simulink model "Vizualize_Measurement"  (R2018b)
settings: Solver=VariableStepAuto  StartTime=0  StopTime=(31+29+31+30+31+30+31+14)*24*3600  RelTol=1e-3  EnableMultiTasking=on
libraries: carnot x16
settings Model: SimulationMode=accelerator  Creator=U_13.adm_zivi  LastModifiedBy=drhf
settings DataIOCC: SaveFormat=Array  SignalLoggingSaveFormat=ModelDataLogs  SaveOutput=off  SignalLogging=off  SaveTime=off
settings OptimizationCC: ExpressionDepthLimit=2147483647  LifeSpan=inf
settings DebuggingCC: UnderspecifiedInitializationDetection=Classic  MergeDetectMultiDrivingBlocksExec=none  SolverPrmCheckMsg=warning  FcnCallInpInsideContextMsg=warning  StateNameClashWarn=warning  SFUnexpectedBacktrackingDiag=warning  SFNoUnconditionalDefaultTransitionDiag=warning  SFExecutionAtInitializationDiag=none
settings HardwareCC: ProdBitPerPointer=32  ProdBitPerSizeT=32  ProdBitPerPtrDiffT=32  ProdLargestAtomicFloat=None  ProdIntDivRoundTo=Undefined  ProdEndianess=Unspecified  ProdWordSize=32  ProdHWDeviceType=32-bit Generic
settings ModelReferenceCC: PropagateSignalLabelsOutOfModel=off
settings SFSimCC: SimUseLocalCustomCode=off
settings RTWCC: RTWUseLocalCustomCode=off
settings CodeAppCC: StateflowObjectComments=on
settings GRTTargetCC: TargetLangStandard=C89/C90 (ANSI)  GeneratePreprocessorConditionals=Disable all  CombineOutputUpdateFcns=off  GRTInterface=on
settings ConfigComp: CovMetricSettings=dw  CovHtmlReporting=on  CovSaveCumulativeToWorkspaceVar=on  CovSaveSingleToWorkspaceVar=on  CovExternalEMLEnable=off

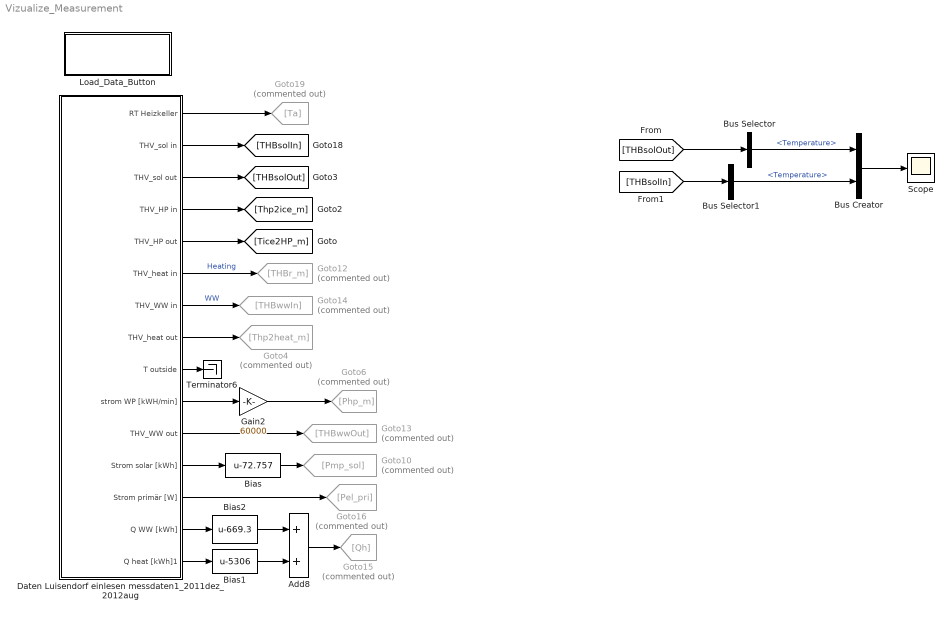
== system Vizualize_Measurement ==
  Add8 : Sum
  Bias : Bias  Bias=-72.757
  Bias1 : Bias  Bias=-5306
  Bias2 : Bias  Bias=-669.3
  Bus Creator : BusCreator  Inputs=2
  Bus Selector : BusSelector  OutputSignals=Temperature
  Bus Selector1 : BusSelector  OutputSignals=Temperature
  Daten Luisendorf einlesen messdaten1_2011dez_2012aug : Subsystem
  Gain2 : Gain  Gain=60000
  Goto10 : Goto  Commented=on  GotoTag=Pmp_sol
  Goto12 : Goto  Commented=on  GotoTag=THBr_m
  Goto13 : Goto  Commented=on  GotoTag=THBwwOut
  Goto14 : Goto  Commented=on  GotoTag=THBwwIn
  Goto15 : Goto  Commented=on  GotoTag=Qh
  Goto16 : Goto  Commented=on  GotoTag=Pel_pri
  Goto19 : Goto  Commented=on  GotoTag=Ta
  Goto4 : Goto  Commented=on  GotoTag=Thp2heat_m
  Goto6 : Goto  Commented=on  GotoTag=Php_m
  Load_Data_Button : Subsystem
      settings: OpenFcn=|
      | [filename, pathname, filterindex] = ...
      |    uigetfile( {'*.mat','MAT-files (*.mat)'; ...
      |    '*.*',  'All Files (*.*)'},  'Pick a data file');
      | 
      | if (filterindex > 0)
      |    load(filename)
      | end
      mask Display: disp('double click \nto load data')
  Scope : Scope
  Terminator6 : Terminator
  wires:
  Daten Luisendorf einlesen messdaten1_2011dez_2012aug/5(THV_HP out) -> [Tice2HP_m]
  Bus Creator/1 -> Scope/1
  Daten Luisendorf einlesen messdaten1_2011dez_2012aug/6(THV_heat in) -> Goto12/1  "Heating"
  Daten Luisendorf einlesen messdaten1_2011dez_2012aug/7(THV_WW in) -> Goto14/1  "WW"
  Daten Luisendorf einlesen messdaten1_2011dez_2012aug/4(THV_HP in) -> [Thp2ice_m]
  Daten Luisendorf einlesen messdaten1_2011dez_2012aug/10(strom WP [kWH/min]) -> Gain2/1
  Daten Luisendorf einlesen messdaten1_2011dez_2012aug/8(THV_heat out) -> Goto4/1
  Daten Luisendorf einlesen messdaten1_2011dez_2012aug/11(THV_WW out) -> Goto13/1
  Daten Luisendorf einlesen messdaten1_2011dez_2012aug/12(Strom solar [kWh]) -> Bias/1
  Bias2/1 -> Add8/1
  Daten Luisendorf einlesen messdaten1_2011dez_2012aug/14(Q WW [kWh]) -> Bias2/1
  Daten Luisendorf einlesen messdaten1_2011dez_2012aug/15(Q heat [kWh]1) -> Bias1/1
  Daten Luisendorf einlesen messdaten1_2011dez_2012aug/9(T outside) -> Terminator6/1
  Daten Luisendorf einlesen messdaten1_2011dez_2012aug/3(THV_sol out) -> [THBsolOut]
  Gain2/1 -> Goto6/1
  Bias/1 -> Goto10/1
  Bias1/1 -> Add8/2
  Add8/1 -> Goto15/1
  Daten Luisendorf einlesen messdaten1_2011dez_2012aug/13(Strom primär [W]) -> Goto16/1
  Daten Luisendorf einlesen messdaten1_2011dez_2012aug/2(THV_sol in) -> [THBsolIn]
  Daten Luisendorf einlesen messdaten1_2011dez_2012aug/1(RT Heizkeller) -> Goto19/1
  [THBsolOut] -> Bus Selector/1
  [THBsolIn] -> Bus Selector1/1
  Bus Selector/1 -> Bus Creator/1  "<Temperature>"
  Bus Selector1/1 -> Bus Creator/2  "<Temperature>"

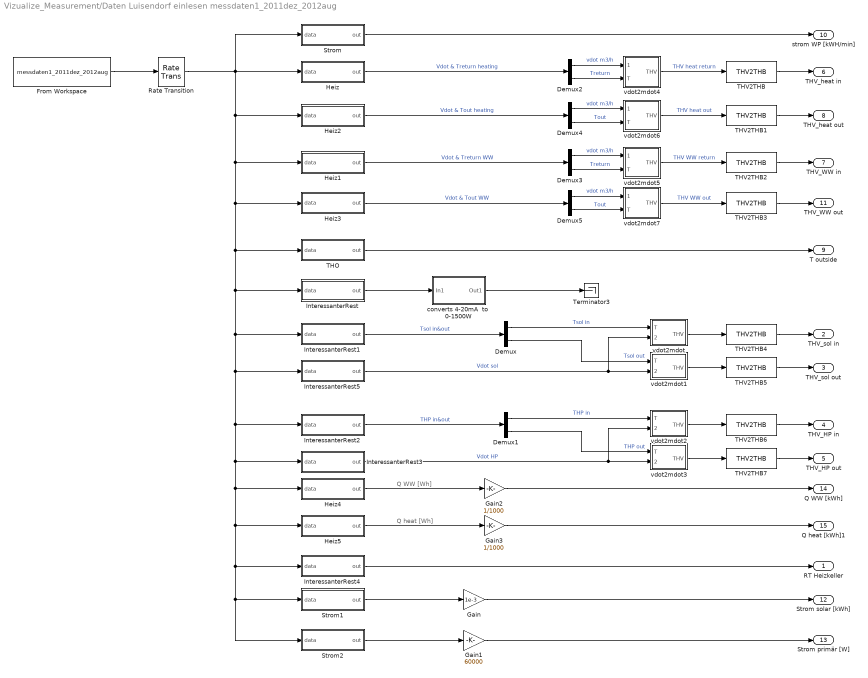
== system Vizualize_Measurement/Daten Luisendorf einlesen messdaten1_2011dez_2012aug ==
  note: Q WW [Wh]
  note: Q heat [Wh]
  Demux{,1..5} (6 alike) : Demux  Outputs=2
  From Workspace : FromWorkspace  VariableName=messdaten1_2011dez_2012aug  SampleTime=60  Interpolate=off  OutputAfterFinalValue=Holding final value
  Gain : Gain  Gain=1e-3
  Gain1 : Gain  Gain=60000
  Gain2 : Gain  Gain=1/1000
  Gain3 : Gain  Gain=1/1000
  Heiz : Subsystem  mask(Selector Messdaten Viessmann){a1=off, a2=off, a3=on, a4=off, a5=on, a6=off, a7=off, a8=off, a9=off, a10=off}
      mask prompts: a1 "Heizkreis_Wh [NONE]"; a2 "Heizkreis_m3 [NONE]"; a3 "Heizkreis_m3/h [NONE]"; a4 "Heizkreis_Tflow [NONE]"; a5 "Heizkreis_Treturn [NONE]"; a6 "TWW+Zirkulation_Wh [NONE]"; a7 "TWW+Zirkulation_m3 [NONE]"; a8 "TWW+Zirkulation_m3/h [NONE]"; a9 "TWW+Zirkulation_Tflow [NONE]"; a10 "TWW+Zirkulation_Treturn [NONE]"
      mask help:
      | Wählt die Messdaten der Viessmann Eisspeicher Anlage aus.
      | Daten der Messungen:
      | Dezember 2011 - August 2012
      mask init:
      | v=[];
      | if (a1)  v = [4];     end
      | if (a2)  v = [v 5];     end
      | if (a3)  v = [v 6];    end
      | if (a4)  v = [v 7];    end
      | if (a5)  v = [v 8];    end
      | if (a6)  v = [v 29];    end
      | if (a7)  v = [v 30];    end
      | if (a8)  v = [v 31];    end
      | if (a9)  v = [v 32];    end
      | if (a10)  v = [v 33];    end
      | if (~numel(v)) v = [6]; end
  Heiz1 : Subsystem  mask(Selector Messdaten Viessmann){a1=off, a2=off, a3=off, a4=off, a5=off, a6=off, a7=off, a8=on, a9=off, a10=on}
      mask prompts: a1 "Heizkreis_Wh [NONE]"; a2 "Heizkreis_m3 [NONE]"; a3 "Heizkreis_m3/h [NONE]"; a4 "Heizkreis_Tflow [NONE]"; a5 "Heizkreis_Treturn [NONE]"; a6 "TWW+Zirkulation_Wh [NONE]"; a7 "TWW+Zirkulation_m3 [NONE]"; a8 "TWW+Zirkulation_m3/h [NONE]"; a9 "TWW+Zirkulation_Tflow [NONE]"; a10 "TWW+Zirkulation_Treturn [NONE]"
      mask help:
      | Wählt die Messdaten der Viessmann Eisspeicher Anlage aus.
      | Daten der Messungen:
      | Dezember 2011 - August 2012
      mask init: same as Vizualize_Measurement/Daten Luisendorf einlesen messdaten1_2011dez_2012aug/Heiz
  Heiz2 : Subsystem  mask(Selector Messdaten Viessmann){a1=off, a2=off, a3=on, a4=on, a5=off, a6=off, a7=off, a8=off, a9=off, a10=off}
      mask prompts: a1 "Heizkreis_Wh [NONE]"; a2 "Heizkreis_m3 [NONE]"; a3 "Heizkreis_m3/h [NONE]"; a4 "Heizkreis_Tflow [NONE]"; a5 "Heizkreis_Treturn [NONE]"; a6 "TWW+Zirkulation_Wh [NONE]"; a7 "TWW+Zirkulation_m3 [NONE]"; a8 "TWW+Zirkulation_m3/h [NONE]"; a9 "TWW+Zirkulation_Tflow [NONE]"; a10 "TWW+Zirkulation_Treturn [NONE]"
      mask help:
      | Wählt die Messdaten der Viessmann Eisspeicher Anlage aus.
      | Daten der Messungen:
      | Dezember 2011 - August 2012
      mask init: same as Vizualize_Measurement/Daten Luisendorf einlesen messdaten1_2011dez_2012aug/Heiz
  Heiz3 : Subsystem  mask(Selector Messdaten Viessmann){a1=off, a2=off, a3=off, a4=off, a5=off, a6=off, a7=off, a8=on, a9=on, a10=off}
      mask prompts: a1 "Heizkreis_Wh [NONE]"; a2 "Heizkreis_m3 [NONE]"; a3 "Heizkreis_m3/h [NONE]"; a4 "Heizkreis_Tflow [NONE]"; a5 "Heizkreis_Treturn [NONE]"; a6 "TWW+Zirkulation_Wh [NONE]"; a7 "TWW+Zirkulation_m3 [NONE]"; a8 "TWW+Zirkulation_m3/h [NONE]"; a9 "TWW+Zirkulation_Tflow [NONE]"; a10 "TWW+Zirkulation_Treturn [NONE]"
      mask help:
      | Wählt die Messdaten der Viessmann Eisspeicher Anlage aus.
      | Daten der Messungen:
      | Dezember 2011 - August 2012
      mask init: same as Vizualize_Measurement/Daten Luisendorf einlesen messdaten1_2011dez_2012aug/Heiz
  Heiz4 : Subsystem  mask(Selector Messdaten Viessmann){a1=off, a2=off, a3=off, a4=off, a5=off, a6=on, a7=off, a8=off, a9=off, a10=off}
      mask prompts: a1 "Heizkreis_Wh [NONE]"; a2 "Heizkreis_m3 [NONE]"; a3 "Heizkreis_m3/h [NONE]"; a4 "Heizkreis_Tflow [NONE]"; a5 "Heizkreis_Treturn [NONE]"; a6 "TWW+Zirkulation_Wh [NONE]"; a7 "TWW+Zirkulation_m3 [NONE]"; a8 "TWW+Zirkulation_m3/h [NONE]"; a9 "TWW+Zirkulation_Tflow [NONE]"; a10 "TWW+Zirkulation_Treturn [NONE]"
      mask help:
      | Wählt die Messdaten der Viessmann Eisspeicher Anlage aus.
      | Daten der Messungen:
      | Dezember 2011 - August 2012
      mask init: same as Vizualize_Measurement/Daten Luisendorf einlesen messdaten1_2011dez_2012aug/Heiz
  Heiz5 : Subsystem  mask(Selector Messdaten Viessmann){a1=on, a2=off, a3=off, a4=off, a5=off, a6=off, a7=off, a8=off, a9=off, a10=off}
      mask prompts: a1 "Heizkreis_Wh [NONE]"; a2 "Heizkreis_m3 [NONE]"; a3 "Heizkreis_m3/h [NONE]"; a4 "Heizkreis_Tflow [NONE]"; a5 "Heizkreis_Treturn [NONE]"; a6 "TWW+Zirkulation_Wh [NONE]"; a7 "TWW+Zirkulation_m3 [NONE]"; a8 "TWW+Zirkulation_m3/h [NONE]"; a9 "TWW+Zirkulation_Tflow [NONE]"; a10 "TWW+Zirkulation_Treturn [NONE]"
      mask help:
      | Wählt die Messdaten der Viessmann Eisspeicher Anlage aus.
      | Daten der Messungen:
      | Dezember 2011 - August 2012
      mask init: same as Vizualize_Measurement/Daten Luisendorf einlesen messdaten1_2011dez_2012aug/Heiz
  InteressanterRest : Subsystem  mask(Selector Messdaten Viessmann){a1=on, a2=off, a3=off, a4=off, a5=off, a6=off, a7=off, a8=off, a9=off, a10=off, a11=off, a12=off, a13=off, a14=off}
      mask prompts: a1 "Einstrahlung [Ampere 4-20mA=0-1500W]"; a2 "Resol  Sol-Eis VL [Celsius]"; a3 "Resol Eis-WP [m^3]"; a4 "Resol Eis-WP RL [Celsius]"; a5 "Resol Eis-WP VL [Celsius]"; a6 "Resol Sol-Eis [m^3]"; a7 "Resol Sol-Eis RL [Celsius]"; a8 "Resol Sol-WP [m^3]"; a9 "Resol Sol-WP RL [Celsius]"; a10 "Resol Sol-WP VL [Celsius]"; a11 "RT Heizkeller [Celsius]"; a12 "Ventil R2_UmschKol [Volt]"; a13 "Ventil_R3_SolPumpe [Volt]"; a14 "Ventil_R4_UmschSpe [Volt]"
      mask help:
      | Wählt die Messdaten der Viessmann Eisspeicher Anlage aus.
      | Daten der Messungen:
      | Dezember 2011 - August 2012
      mask init:
      | v=[];
      | if (a1)  v = [3];     end
      | if (a2)  v = [v 9];     end
      | if (a3)  v = [v 10];    end
      | if (a4)  v = [v 11];    end
      | if (a5)  v = [v 12];    end
      | if (a6)  v = [v 13];    end
      | if (a7)  v = [v 14];     end
      | if (a8)  v = [v 15];     end
      | if (a9)  v = [v 16];    end
      | if (a10)  v = [v 17];    end
      | if (a11)  v = [v 18];    end
      | if (a12)  v = [v 34];    end
      | if (a13)  v = [v 35];     end
      | if (a14)  v = [v 36];     end
      | if (~numel(v)) v = [6]; end
  InteressanterRest1 : Subsystem  mask(Selector Messdaten Viessmann){a1=off, a2=on, a3=off, a4=off, a5=off, a6=off, a7=on, a8=off, a9=off, a10=off, a11=off, a12=off, a13=off, a14=off}
      mask prompts: a1 "Einstrahlung [Ampere 4-20mA=0-1500W]"; a2 "Resol  Sol-Eis VL [Celsius]"; a3 "Resol Eis-WP [m^3]"; a4 "Resol Eis-WP RL [Celsius]"; a5 "Resol Eis-WP VL [Celsius]"; a6 "Resol Sol-Eis [m^3]"; a7 "Resol Sol-Eis RL [Celsius]"; a8 "Resol Sol-WP [m^3]"; a9 "Resol Sol-WP RL [Celsius]"; a10 "Resol Sol-WP VL [Celsius]"; a11 "RT Heizkeller [Celsius]"; a12 "Ventil R2_UmschKol [Volt]"; a13 "Ventil_R3_SolPumpe [Volt]"; a14 "Ventil_R4_UmschSpe [Volt]"
      mask help:
      | Wählt die Messdaten der Viessmann Eisspeicher Anlage aus.
      | Daten der Messungen:
      | Dezember 2011 - August 2012
      mask init: same as Vizualize_Measurement/Daten Luisendorf einlesen messdaten1_2011dez_2012aug/InteressanterRest
  InteressanterRest2 : Subsystem  mask(Selector Messdaten Viessmann){a1=off, a2=off, a3=off, a4=on, a5=on, a6=off, a7=off, a8=off, a9=off, a10=off, a11=off, a12=off, a13=off, a14=off}
      mask prompts: a1 "Einstrahlung [Ampere 4-20mA=0-1500W]"; a2 "Resol  Sol-Eis VL [Celsius]"; a3 "Resol Eis-WP [m^3]"; a4 "Resol Eis-WP RL [Celsius]"; a5 "Resol Eis-WP VL [Celsius]"; a6 "Resol Sol-Eis [m^3]"; a7 "Resol Sol-Eis RL [Celsius]"; a8 "Resol Sol-WP [m^3]"; a9 "Resol Sol-WP RL [Celsius]"; a10 "Resol Sol-WP VL [Celsius]"; a11 "RT Heizkeller [Celsius]"; a12 "Ventil R2_UmschKol [Volt]"; a13 "Ventil_R3_SolPumpe [Volt]"; a14 "Ventil_R4_UmschSpe [Volt]"
      mask help:
      | Wählt die Messdaten der Viessmann Eisspeicher Anlage aus.
      | Daten der Messungen:
      | Dezember 2011 - August 2012
      mask init: same as Vizualize_Measurement/Daten Luisendorf einlesen messdaten1_2011dez_2012aug/InteressanterRest
  InteressanterRest3 : Subsystem  mask(Selector Messdaten Viessmann){a1=off, a2=off, a3=on, a4=off, a5=off, a6=off, a7=off, a8=off, a9=off, a10=off, a11=off, a12=off, a13=off, a14=off}
      mask prompts: a1 "Einstrahlung [Ampere 4-20mA=0-1500W]"; a2 "Resol  Sol-Eis VL [Celsius]"; a3 "Resol Eis-WP [m^3]"; a4 "Resol Eis-WP RL [Celsius]"; a5 "Resol Eis-WP VL [Celsius]"; a6 "Resol Sol-Eis [m^3]"; a7 "Resol Sol-Eis RL [Celsius]"; a8 "Resol Sol-WP [m^3]"; a9 "Resol Sol-WP RL [Celsius]"; a10 "Resol Sol-WP VL [Celsius]"; a11 "RT Heizkeller [Celsius]"; a12 "Ventil R2_UmschKol [Volt]"; a13 "Ventil_R3_SolPumpe [Volt]"; a14 "Ventil_R4_UmschSpe [Volt]"
      mask help:
      | Wählt die Messdaten der Viessmann Eisspeicher Anlage aus.
      | Daten der Messungen:
      | Dezember 2011 - August 2012
      mask init: same as Vizualize_Measurement/Daten Luisendorf einlesen messdaten1_2011dez_2012aug/InteressanterRest
  InteressanterRest4 : Subsystem  mask(Selector Messdaten Viessmann){a1=off, a2=off, a3=off, a4=off, a5=off, a6=off, a7=off, a8=off, a9=off, a10=off, a11=on, a12=off, a13=off, a14=off}
      mask prompts: a1 "Einstrahlung [Ampere 4-20mA=0-1500W]"; a2 "Resol  Sol-Eis VL [Celsius]"; a3 "Resol Eis-WP [m^3]"; a4 "Resol Eis-WP RL [Celsius]"; a5 "Resol Eis-WP VL [Celsius]"; a6 "Resol Sol-Eis [m^3]"; a7 "Resol Sol-Eis RL [Celsius]"; a8 "Resol Sol-WP [m^3]"; a9 "Resol Sol-WP RL [Celsius]"; a10 "Resol Sol-WP VL [Celsius]"; a11 "RT Heizkeller [Celsius]"; a12 "Ventil R2_UmschKol [Volt]"; a13 "Ventil_R3_SolPumpe [Volt]"; a14 "Ventil_R4_UmschSpe [Volt]"
      mask help:
      | Wählt die Messdaten der Viessmann Eisspeicher Anlage aus.
      | Daten der Messungen:
      | Dezember 2011 - August 2012
      mask init: same as Vizualize_Measurement/Daten Luisendorf einlesen messdaten1_2011dez_2012aug/InteressanterRest
  InteressanterRest5 : Subsystem  mask(Selector Messdaten Viessmann){a1=off, a2=off, a3=off, a4=off, a5=off, a6=on, a7=off, a8=off, a9=off, a10=off, a11=off, a12=off, a13=off, a14=off}
      mask prompts: a1 "Einstrahlung [Ampere 4-20mA=0-1500W]"; a2 "Resol  Sol-Eis VL [Celsius]"; a3 "Resol Eis-WP [m^3]"; a4 "Resol Eis-WP RL [Celsius]"; a5 "Resol Eis-WP VL [Celsius]"; a6 "Resol Sol-Eis [m^3]"; a7 "Resol Sol-Eis RL [Celsius]"; a8 "Resol Sol-WP [m^3]"; a9 "Resol Sol-WP RL [Celsius]"; a10 "Resol Sol-WP VL [Celsius]"; a11 "RT Heizkeller [Celsius]"; a12 "Ventil R2_UmschKol [Volt]"; a13 "Ventil_R3_SolPumpe [Volt]"; a14 "Ventil_R4_UmschSpe [Volt]"
      mask help:
      | Wählt die Messdaten der Viessmann Eisspeicher Anlage aus.
      | Daten der Messungen:
      | Dezember 2011 - August 2012
      mask init: same as Vizualize_Measurement/Daten Luisendorf einlesen messdaten1_2011dez_2012aug/InteressanterRest
  Rate Transition : RateTransition
  Strom : Subsystem  mask(Selector Messdaten Viessmann){a1=off, a2=on, a3=off, a4=off, a5=off, a6=off}
      mask prompts: a1 "Drehstrom E-Heizst [kWh]"; a2 "Drestrom WP [kWh]"; a3 "Strom Primärpumpe [kWh]"; a4 "Strom Regelung [kWh]"; a5 "Strom Sekundärpump [kWh]"; a6 "Strom Solarstation [NONE]"
      mask help:
      | Wählt die Messdaten der Viessmann Eisspeicher Anlage aus.
      | Daten der Messungen:
      | Dezember 2011 - August 2012
      mask init:
      | v=[];
      | if (a1)  v = [1];     end
      | if (a2)  v = [v 2];     end
      | if (a3)  v = [v 19];    end
      | if (a4)  v = [v 20];    end
      | if (a5)  v = [v 21];    end
      | if (a6)  v = [v 22];    end
      | if (~numel(v)) v = [6]; end
  Strom1 : Subsystem  mask(Selector Messdaten Viessmann){a1=off, a2=off, a3=off, a4=off, a5=off, a6=on}
      mask prompts: a1 "Drehstrom E-Heizst [kWh]"; a2 "Drestrom WP [kWh]"; a3 "Strom Primärpumpe [kWh]"; a4 "Strom Regelung [kWh]"; a5 "Strom Sekundärpump [kWh]"; a6 "Strom Solarstation [NONE]"
      mask help:
      | Wählt die Messdaten der Viessmann Eisspeicher Anlage aus.
      | Daten der Messungen:
      | Dezember 2011 - August 2012
      mask init:
      | v=[];
      | if (a1)  v = [1];     end
      | if (a2)  v = [v 2];     end
      | if (a3)  v = [v 19];    end
      | if (a4)  v = [v 20];    end
      | if (a5)  v = [v 21];    end
      | if (a6)  v = [v 22];    end
      | if (~numel(v)) v = [6]; end
  Strom2 : Subsystem  mask(Selector Messdaten Viessmann){a1=off, a2=off, a3=on, a4=off, a5=off, a6=off}
      mask prompts: a1 "Drehstrom E-Heizst [kWh]"; a2 "Drestrom WP [kWh]"; a3 "Strom Primärpumpe [kWh]"; a4 "Strom Regelung [kWh]"; a5 "Strom Sekundärpump [kWh]"; a6 "Strom Solarstation [NONE]"
      mask help:
      | Wählt die Messdaten der Viessmann Eisspeicher Anlage aus.
      | Daten der Messungen:
      | Dezember 2011 - August 2012
      mask init:
      | v=[];
      | if (a1)  v = [1];     end
      | if (a2)  v = [v 2];     end
      | if (a3)  v = [v 19];    end
      | if (a4)  v = [v 20];    end
      | if (a5)  v = [v 21];    end
      | if (a6)  v = [v 22];    end
      | if (~numel(v)) v = [6]; end
  THO : Subsystem  mask(Selector Messdaten Viessmann){a1=off, a2=off, a3=off, a4=on, a5=off, a6=off}
      mask prompts: a1 "THO_rhoinst [NONE]"; a2 "THO_rhomax [NONE]"; a3 "THO_rhomin [NONE]"; a4 "THO_Tinst [NONE]"; a5 "THO_Tmax [NONE]"; a6 "THO_Tmin [NONE]"
      mask help:
      | Wählt die Messdaten der Viessmann Eisspeicher Anlage aus.
      | Daten der Messungen:
      | Dezember 2011 - August 2012
      mask init:
      | v=[];
      | if (a1)  v = [23];     end
      | if (a2)  v = [v 24];     end
      | if (a3)  v = [v 25];    end
      | if (a4)  v = [v 26];    end
      | if (a5)  v = [v 27];    end
      | if (a6)  v = [v 28];    end
      | if (~numel(v)) v = [6]; end
  THV2THB{,1..7} (8 alike) : carnot/Toolbox/THV2THB
      settings: SourceProductName=Carnot
  Terminator3 : Terminator
  converts 4-20mA  to  0-1500W : Subsystem
  vdot2mdot : Subsystem  mask(create THV){p=1e5, fluid=water_glycol_mix, mix=0.5, dia=0.025}
      mask prompts: p "pressure [Pa]"; mix "fluid mixture [0..1]"; dia "diameter [m]"
      mask help: Block to create a THV vector with the variable input T and mdot. The other value can be set as constants in the mask.
      mask init:
      | mix = min(1, max(0, mix));
      | dia = max(dia, 0.001);
      mask Help: eval('man (''create_THV'')')
      mask TypeOptions fluid: water | air | cotton_oil | silicone_oil | water_glycol_mix
  vdot2mdot1 : Subsystem  mask(create THV){p=1e5, fluid=water_glycol_mix, mix=0.5, dia=0.025}
      mask prompts: p "pressure [Pa]"; mix "fluid mixture [0..1]"; dia "diameter [m]"
      mask help: Block to create a THV vector with the variable input T and mdot. The other value can be set as constants in the mask.
      mask init:
      | mix = min(1, max(0, mix));
      | dia = max(dia, 0.001);
      mask Help: eval('man (''create_THV'')')
      mask TypeOptions fluid: water | air | cotton_oil | silicone_oil | water_glycol_mix
  vdot2mdot2 : Subsystem  mask(create THV){p=1e5, fluid=water_glycol_mix, mix=0.5, dia=0.025}
      mask prompts: p "pressure [Pa]"; mix "fluid mixture [0..1]"; dia "diameter [m]"
      mask help: Block to create a THV vector with the variable input T and mdot. The other value can be set as constants in the mask.
      mask init:
      | mix = min(1, max(0, mix));
      | dia = max(dia, 0.001);
      mask Help: eval('man (''create_THV'')')
      mask TypeOptions fluid: water | air | cotton_oil | silicone_oil | water_glycol_mix
  vdot2mdot3 : Subsystem  mask(create THV){p=1e5, fluid=water_glycol_mix, mix=0.5, dia=0.025}
      mask prompts: p "pressure [Pa]"; mix "fluid mixture [0..1]"; dia "diameter [m]"
      mask help: Block to create a THV vector with the variable input T and mdot. The other value can be set as constants in the mask.
      mask init:
      | mix = min(1, max(0, mix));
      | dia = max(dia, 0.001);
      mask Help: eval('man (''create_THV'')')
      mask TypeOptions fluid: water | air | cotton_oil | silicone_oil | water_glycol_mix
  vdot2mdot4 : Subsystem  mask(create THV){p=1e5, fluid=water, mix=0, dia=0.025}
      mask prompts: p "pressure [Pa]"; mix "fluid mixture [0..1]"; dia "diameter [m]"
      mask help: Block to create a THV vector with the variable input T and mdot. The other value can be set as constants in the mask.
      mask init:
      | mix = min(1, max(0, mix));
      | dia = max(dia, 0.001);
      mask Help: eval('man (''create_THV'')')
      mask TypeOptions fluid: water | air | cotton_oil | silicone_oil | water_glycol_mix
  vdot2mdot5 : Subsystem  mask(create THV){p=1e5, fluid=water, mix=0, dia=0.025}
      mask prompts: p "pressure [Pa]"; mix "fluid mixture [0..1]"; dia "diameter [m]"
      mask help: Block to create a THV vector with the variable input T and mdot. The other value can be set as constants in the mask.
      mask init:
      | mix = min(1, max(0, mix));
      | dia = max(dia, 0.001);
      mask Help: eval('man (''create_THV'')')
      mask TypeOptions fluid: water | air | cotton_oil | silicone_oil | water_glycol_mix
  vdot2mdot6 : Subsystem  mask(create THV){p=1e5, fluid=water, mix=0, dia=0.025}
      mask prompts: p "pressure [Pa]"; mix "fluid mixture [0..1]"; dia "diameter [m]"
      mask help: Block to create a THV vector with the variable input T and mdot. The other value can be set as constants in the mask.
      mask init:
      | mix = min(1, max(0, mix));
      | dia = max(dia, 0.001);
      mask Help: eval('man (''create_THV'')')
      mask TypeOptions fluid: water | air | cotton_oil | silicone_oil | water_glycol_mix
  vdot2mdot7 : Subsystem  mask(create THV){p=1e5, fluid=water, mix=0, dia=0.025}
      mask prompts: p "pressure [Pa]"; mix "fluid mixture [0..1]"; dia "diameter [m]"
      mask help: Block to create a THV vector with the variable input T and mdot. The other value can be set as constants in the mask.
      mask init:
      | mix = min(1, max(0, mix));
      | dia = max(dia, 0.001);
      mask Help: eval('man (''create_THV'')')
      mask TypeOptions fluid: water | air | cotton_oil | silicone_oil | water_glycol_mix
  RT Heizkeller : Outport
  THV_sol in : Outport  Port=2
  THV_sol out : Outport  Port=3
  THV_HP in : Outport  Port=4
  THV_HP out : Outport  Port=5
  THV_heat in : Outport  Port=6
  THV_WW in : Outport  Port=7
  THV_heat out : Outport  Port=8
  T outside : Outport  Port=9
  strom WP [kWH/min] : Outport  Port=10
  THV_WW out : Outport  Port=11
  Strom solar [kWh] : Outport  Port=12
  Strom primär [W] : Outport  Port=13
  Q WW [kWh] : Outport  Port=14
  Q heat [kWh]1 : Outport  Port=15
  wires:
  THO/1(out) -> T outside/1
  Heiz/1(out) -> Demux2/1  "Vdot & Treturn heating"
  converts 4-20mA  to  0-1500W/1(Out1) -> Terminator3/1
  InteressanterRest/1(out) -> converts 4-20mA  to  0-1500W/1(In1)
  Strom/1(out) -> strom WP [kWH/min]/1
  From Workspace/1 -> Rate Transition/1
  InteressanterRest1/1(out) -> Demux/1  "Tsol in&out"
  InteressanterRest2/1(out) -> Demux1/1  "THP in&out"
  InteressanterRest3/1(out) -> vdot2mdot3/2(vdot), vdot2mdot2/2(vdot)  "Vdot HP"
  InteressanterRest4/1(out) -> RT Heizkeller/1
  InteressanterRest5/1(out) -> vdot2mdot1/2(vdot), vdot2mdot/2(vdot)  "Vdot sol"
  Demux/1 -> vdot2mdot/1(T)  "Tsol in"
  Demux/2 -> vdot2mdot1/1(T)  "Tsol out"
  vdot2mdot/1(THV) -> THV2THB4/1
  vdot2mdot1/1(THV) -> THV2THB5/1
  Demux1/1 -> vdot2mdot2/1(T)  "THP in"
  Demux1/2 -> vdot2mdot3/1(T)  "THP out"
  vdot2mdot2/1(THV) -> THV2THB6/1
  vdot2mdot3/1(THV) -> THV2THB7/1
  Demux2/1 -> vdot2mdot4/1(vdot)  "vdot m3/h"
  Demux2/2 -> vdot2mdot4/2(T)  "Treturn"
  vdot2mdot4/1(THV) -> THV2THB/1  "THV heat return"
  Heiz1/1(out) -> Demux3/1  "Vdot & Treturn WW"
  Demux3/1 -> vdot2mdot5/1(vdot)  "vdot m3/h"
  Demux3/2 -> vdot2mdot5/2(T)  "Treturn"
  vdot2mdot5/1(THV) -> THV2THB2/1  "THV WW return"
  Heiz2/1(out) -> Demux4/1  "Vdot & Tout heating"
  Demux4/1 -> vdot2mdot6/1(vdot)  "vdot m3/h"
  Demux4/2 -> vdot2mdot6/2(T)  "Tout"
  vdot2mdot6/1(THV) -> THV2THB1/1  "THV heat out"
  Heiz3/1(out) -> Demux5/1  "Vdot & Tout WW"
  Demux5/1 -> vdot2mdot7/1(vdot)  "vdot m3/h"
  Demux5/2 -> vdot2mdot7/2(T)  "Tout"
  vdot2mdot7/1(THV) -> THV2THB3/1  "THV WW out"
  Strom1/1(out) -> Gain/1
  Gain/1 -> Strom solar [kWh]/1
  Strom2/1(out) -> Gain1/1
  Gain1/1 -> Strom primär [W]/1
  Heiz4/1(out) -> Gain2/1
  Gain2/1 -> Q WW [kWh]/1
  Heiz5/1(out) -> Gain3/1
  Gain3/1 -> Q heat [kWh]1/1
  THV2THB/1 -> THV_heat in/1
  THV2THB1/1 -> THV_heat out/1
  THV2THB2/1 -> THV_WW in/1
  THV2THB3/1 -> THV_WW out/1
  THV2THB4/1 -> THV_sol in/1
  THV2THB5/1 -> THV_sol out/1
  THV2THB6/1 -> THV_HP in/1
  THV2THB7/1 -> THV_HP out/1
  Rate Transition/1 -> Heiz1/1(data), InteressanterRest1/1(data), InteressanterRest2/1(data), InteressanterRest3/1(data), Heiz4/1(data), InteressanterRest4/1(data), Strom1/1(data), Strom2/1(data), Heiz5/1(data), InteressanterRest5/1(data), InteressanterRest/1(data), THO/1(data), Heiz3/1(data), Heiz2/1(data), Strom/1(data), Heiz/1(data)

== system Vizualize_Measurement/Load_Data_Button ==

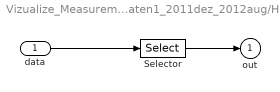
== system Vizualize_Measurement/Daten Luisendorf einlesen messdaten1_2011dez_2012aug/Heiz ==
  data : Inport
  Selector : Selector  InputPortWidth=36  IndexOptions=Index vector (dialog)  Indices=[v]  OutputSizes=1
  out : Outport  InitialOutput=0
  wires:
  data/1 -> Selector/1
  Selector/1 -> out/1

== system Vizualize_Measurement/Daten Luisendorf einlesen messdaten1_2011dez_2012aug/Heiz1 ==
  data : Inport
  Selector : Selector  InputPortWidth=36  IndexOptions=Index vector (dialog)  Indices=[v]  OutputSizes=1
  out : Outport  InitialOutput=0
  wires:
  Selector/1 -> out/1
  data/1 -> Selector/1

== system Vizualize_Measurement/Daten Luisendorf einlesen messdaten1_2011dez_2012aug/Heiz2 ==
  data : Inport
  Selector : Selector  InputPortWidth=36  IndexOptions=Index vector (dialog)  Indices=[v]  OutputSizes=1
  out : Outport  InitialOutput=0
  wires:
  Selector/1 -> out/1
  data/1 -> Selector/1

== system Vizualize_Measurement/Daten Luisendorf einlesen messdaten1_2011dez_2012aug/Heiz3 ==
  data : Inport
  Selector : Selector  InputPortWidth=36  IndexOptions=Index vector (dialog)  Indices=[v]  OutputSizes=1
  out : Outport  InitialOutput=0
  wires:
  data/1 -> Selector/1
  Selector/1 -> out/1

== system Vizualize_Measurement/Daten Luisendorf einlesen messdaten1_2011dez_2012aug/Heiz4 ==
  data : Inport
  Selector : Selector  InputPortWidth=36  IndexOptions=Index vector (dialog)  Indices=[v]  OutputSizes=1
  out : Outport  InitialOutput=0
  wires:
  Selector/1 -> out/1
  data/1 -> Selector/1

== system Vizualize_Measurement/Daten Luisendorf einlesen messdaten1_2011dez_2012aug/Heiz5 ==
  data : Inport
  Selector : Selector  InputPortWidth=36  IndexOptions=Index vector (dialog)  Indices=[v]  OutputSizes=1
  out : Outport  InitialOutput=0
  wires:
  data/1 -> Selector/1
  Selector/1 -> out/1

== system Vizualize_Measurement/Daten Luisendorf einlesen messdaten1_2011dez_2012aug/InteressanterRest ==
  data : Inport
  Selector : Selector  InputPortWidth=36  IndexOptions=Index vector (dialog)  Indices=[v]  OutputSizes=1
  out : Outport  InitialOutput=0
  wires:
  data/1 -> Selector/1
  Selector/1 -> out/1

== system Vizualize_Measurement/Daten Luisendorf einlesen messdaten1_2011dez_2012aug/InteressanterRest1 ==
  data : Inport
  Selector : Selector  InputPortWidth=36  IndexOptions=Index vector (dialog)  Indices=[v]  OutputSizes=1
  out : Outport  InitialOutput=0
  wires:
  Selector/1 -> out/1
  data/1 -> Selector/1

== system Vizualize_Measurement/Daten Luisendorf einlesen messdaten1_2011dez_2012aug/InteressanterRest2 ==
  data : Inport
  Selector : Selector  InputPortWidth=36  IndexOptions=Index vector (dialog)  Indices=[v]  OutputSizes=1
  out : Outport  InitialOutput=0
  wires:
  data/1 -> Selector/1
  Selector/1 -> out/1

== system Vizualize_Measurement/Daten Luisendorf einlesen messdaten1_2011dez_2012aug/InteressanterRest3 ==
  data : Inport
  Selector : Selector  InputPortWidth=36  IndexOptions=Index vector (dialog)  Indices=[v]  OutputSizes=1
  out : Outport  InitialOutput=0
  wires:
  Selector/1 -> out/1
  data/1 -> Selector/1

== system Vizualize_Measurement/Daten Luisendorf einlesen messdaten1_2011dez_2012aug/InteressanterRest4 ==
  data : Inport
  Selector : Selector  InputPortWidth=36  IndexOptions=Index vector (dialog)  Indices=[v]  OutputSizes=1
  out : Outport  InitialOutput=0
  wires:
  data/1 -> Selector/1
  Selector/1 -> out/1

== system Vizualize_Measurement/Daten Luisendorf einlesen messdaten1_2011dez_2012aug/InteressanterRest5 ==
  data : Inport
  Selector : Selector  InputPortWidth=36  IndexOptions=Index vector (dialog)  Indices=[v]  OutputSizes=1
  out : Outport  InitialOutput=0
  wires:
  data/1 -> Selector/1
  Selector/1 -> out/1

== system Vizualize_Measurement/Daten Luisendorf einlesen messdaten1_2011dez_2012aug/Strom ==
  data : Inport
  Selector : Selector  InputPortWidth=36  IndexOptions=Index vector (dialog)  Indices=[v]  OutputSizes=1
  out : Outport  InitialOutput=0
  wires:
  Selector/1 -> out/1
  data/1 -> Selector/1

== system Vizualize_Measurement/Daten Luisendorf einlesen messdaten1_2011dez_2012aug/Strom1 ==
  data : Inport
  Selector : Selector  InputPortWidth=36  IndexOptions=Index vector (dialog)  Indices=[v]  OutputSizes=1
  out : Outport  InitialOutput=0
  wires:
  data/1 -> Selector/1
  Selector/1 -> out/1

== system Vizualize_Measurement/Daten Luisendorf einlesen messdaten1_2011dez_2012aug/Strom2 ==
  data : Inport
  Selector : Selector  InputPortWidth=36  IndexOptions=Index vector (dialog)  Indices=[v]  OutputSizes=1
  out : Outport  InitialOutput=0
  wires:
  Selector/1 -> out/1
  data/1 -> Selector/1

== system Vizualize_Measurement/Daten Luisendorf einlesen messdaten1_2011dez_2012aug/THO ==
  data : Inport
  Selector : Selector  InputPortWidth=36  IndexOptions=Index vector (dialog)  Indices=[v]  OutputSizes=1
  out : Outport  InitialOutput=0
  wires:
  Selector/1 -> out/1
  data/1 -> Selector/1

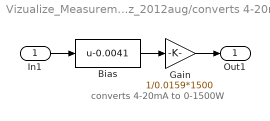
== system Vizualize_Measurement/Daten Luisendorf einlesen messdaten1_2011dez_2012aug/converts 4-20mA  to  0-1500W ==
  note: converts
      | 4-20mA  to  0-1500W
  In1 : Inport
  Bias : Bias  Bias=-0.0041
  Gain : Gain  Gain=1/0.0159*1500
  Out1 : Outport
  wires:
  Gain/1 -> Out1/1
  In1/1 -> Bias/1
  Bias/1 -> Gain/1

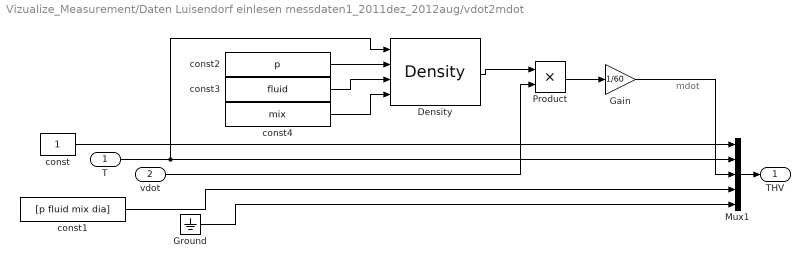
== system Vizualize_Measurement/Daten Luisendorf einlesen messdaten1_2011dez_2012aug/vdot2mdot ==
  note: mdot
  T : Inport
  vdot : Inport  Port=2
  Density : carnot/Basic/Material_Properties/Density  VariantControl=CarlibClassic  INPUTARGUMENTS=state variables (classic)  DEBUGLEVEL=DEBUGLEVEL  MAXTOTALWARNINGS=inf  MAXCONSECUTIVEWARNINGS=inf  WRITETOFILE=0  FILENAME='errors.txt'
      settings: SourceProductName=Carnot
  Gain : Gain  Gain=1/60
  Ground : Ground
  Mux1 : Mux  Inputs=[1 1 1 4 13]
  Product : Product  RndMeth=Zero
  const : Constant
  const1 : Constant  Value=[p fluid mix dia]
  const2 : Constant  Value=p
  const3 : Constant  Value=fluid
  const4 : Constant  Value=mix
  THV : Outport  InitialOutput=0
  wires:
  const1/1 -> Mux1/4
  T/1 -> Density/1, Mux1/2
  Ground/1 -> Mux1/5
  const/1 -> Mux1/1
  Mux1/1 -> THV/1
  const2/1 -> Density/2
  const3/1 -> Density/3
  const4/1 -> Density/4
  Density/1 -> Product/1
  vdot/1 -> Product/2
  Product/1 -> Gain/1
  Gain/1 -> Mux1/3

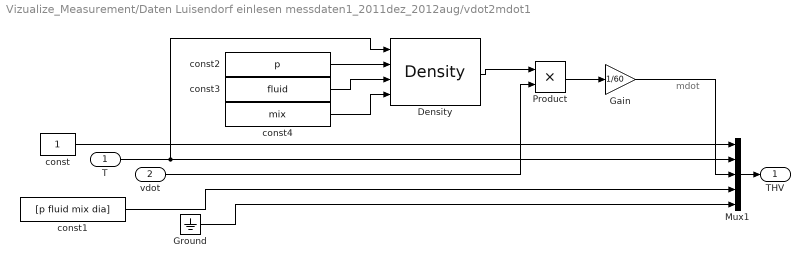
== system Vizualize_Measurement/Daten Luisendorf einlesen messdaten1_2011dez_2012aug/vdot2mdot1 ==
  note: mdot
  T : Inport
  vdot : Inport  Port=2
  Density : carnot/Basic/Material_Properties/Density  VariantControl=CarlibClassic  INPUTARGUMENTS=state variables (classic)  DEBUGLEVEL=DEBUGLEVEL  MAXTOTALWARNINGS=inf  MAXCONSECUTIVEWARNINGS=inf  WRITETOFILE=0  FILENAME='errors.txt'
      settings: SourceProductName=Carnot
  Gain : Gain  Gain=1/60
  Ground : Ground
  Mux1 : Mux  Inputs=[1 1 1 4 13]
  Product : Product  RndMeth=Zero
  const : Constant
  const1 : Constant  Value=[p fluid mix dia]
  const2 : Constant  Value=p
  const3 : Constant  Value=fluid
  const4 : Constant  Value=mix
  THV : Outport  InitialOutput=0
  wires:
  Gain/1 -> Mux1/3
  Product/1 -> Gain/1
  vdot/1 -> Product/2
  Density/1 -> Product/1
  const4/1 -> Density/4
  const3/1 -> Density/3
  const2/1 -> Density/2
  Mux1/1 -> THV/1
  const/1 -> Mux1/1
  Ground/1 -> Mux1/5
  T/1 -> Density/1, Mux1/2
  const1/1 -> Mux1/4

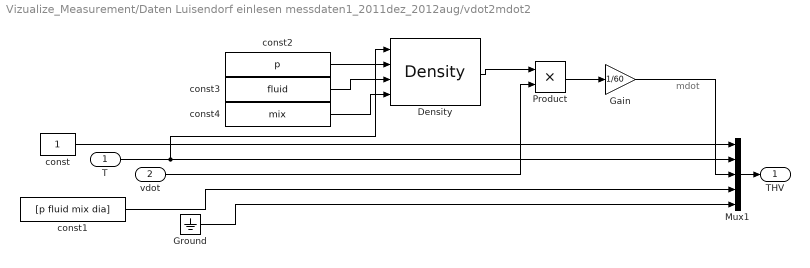
== system Vizualize_Measurement/Daten Luisendorf einlesen messdaten1_2011dez_2012aug/vdot2mdot2 ==
  note: mdot
  T : Inport
  vdot : Inport  Port=2
  Density : carnot/Basic/Material_Properties/Density  VariantControl=CarlibClassic  INPUTARGUMENTS=state variables (classic)  DEBUGLEVEL=DEBUGLEVEL  MAXTOTALWARNINGS=inf  MAXCONSECUTIVEWARNINGS=inf  WRITETOFILE=0  FILENAME='errors.txt'
      settings: SourceProductName=Carnot
  Gain : Gain  Gain=1/60
  Ground : Ground
  Mux1 : Mux  Inputs=[1 1 1 4 13]
  Product : Product  RndMeth=Zero
  const : Constant
  const1 : Constant  Value=[p fluid mix dia]
  const2 : Constant  Value=p
  const3 : Constant  Value=fluid
  const4 : Constant  Value=mix
  THV : Outport  InitialOutput=0
  wires:
  Gain/1 -> Mux1/3
  Product/1 -> Gain/1
  vdot/1 -> Product/2
  Density/1 -> Product/1
  const4/1 -> Density/4
  const3/1 -> Density/3
  const2/1 -> Density/2
  Mux1/1 -> THV/1
  const/1 -> Mux1/1
  Ground/1 -> Mux1/5
  T/1 -> Density/1, Mux1/2
  const1/1 -> Mux1/4

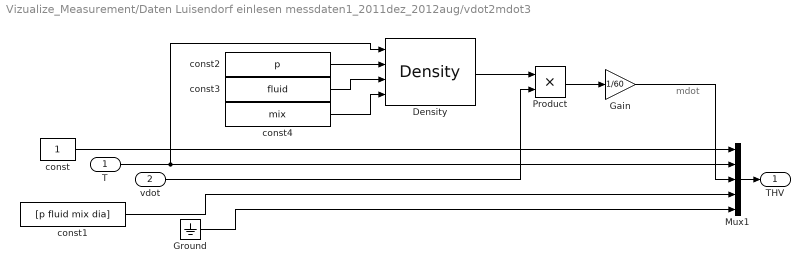
== system Vizualize_Measurement/Daten Luisendorf einlesen messdaten1_2011dez_2012aug/vdot2mdot3 ==
  note: mdot
  T : Inport
  vdot : Inport  Port=2
  Density : carnot/Basic/Material_Properties/Density  VariantControl=CarlibClassic  INPUTARGUMENTS=state variables (classic)  DEBUGLEVEL=DEBUGLEVEL  MAXTOTALWARNINGS=inf  MAXCONSECUTIVEWARNINGS=inf  WRITETOFILE=0  FILENAME='errors.txt'
      settings: SourceProductName=Carnot
  Gain : Gain  Gain=1/60
  Ground : Ground
  Mux1 : Mux  Inputs=[1 1 1 4 13]
  Product : Product  RndMeth=Zero
  const : Constant
  const1 : Constant  Value=[p fluid mix dia]
  const2 : Constant  Value=p
  const3 : Constant  Value=fluid
  const4 : Constant  Value=mix
  THV : Outport  InitialOutput=0
  wires:
  const1/1 -> Mux1/4
  T/1 -> Density/1, Mux1/2
  Ground/1 -> Mux1/5
  const/1 -> Mux1/1
  Mux1/1 -> THV/1
  const2/1 -> Density/2
  const3/1 -> Density/3
  const4/1 -> Density/4
  Density/1 -> Product/1
  vdot/1 -> Product/2
  Product/1 -> Gain/1
  Gain/1 -> Mux1/3

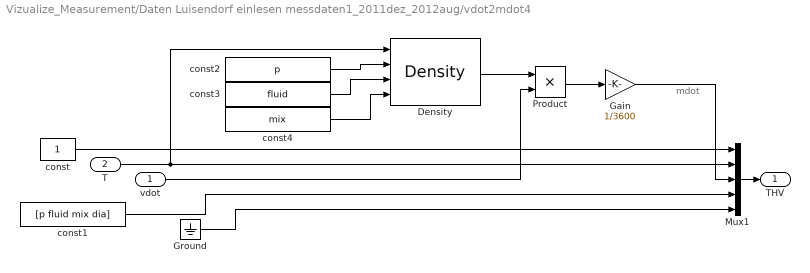
== system Vizualize_Measurement/Daten Luisendorf einlesen messdaten1_2011dez_2012aug/vdot2mdot4 ==
  note: mdot
  vdot : Inport
  T : Inport  Port=2
  Density : carnot/Basic/Material_Properties/Density  VariantControl=CarlibClassic  INPUTARGUMENTS=state variables (classic)  DEBUGLEVEL=DEBUGLEVEL  MAXTOTALWARNINGS=inf  MAXCONSECUTIVEWARNINGS=inf  WRITETOFILE=0  FILENAME='errors.txt'
      settings: SourceProductName=Carnot
  Gain : Gain  Gain=1/3600
  Ground : Ground
  Mux1 : Mux  Inputs=[1 1 1 4 13]
  Product : Product  RndMeth=Zero
  const : Constant
  const1 : Constant  Value=[p fluid mix dia]
  const2 : Constant  Value=p
  const3 : Constant  Value=fluid
  const4 : Constant  Value=mix
  THV : Outport  InitialOutput=0
  wires:
  Product/1 -> Gain/1
  vdot/1 -> Product/2
  Density/1 -> Product/1
  const4/1 -> Density/4
  const3/1 -> Density/3
  const2/1 -> Density/2
  Mux1/1 -> THV/1
  const/1 -> Mux1/1
  Ground/1 -> Mux1/5
  T/1 -> Density/1, Mux1/2
  const1/1 -> Mux1/4
  Gain/1 -> Mux1/3

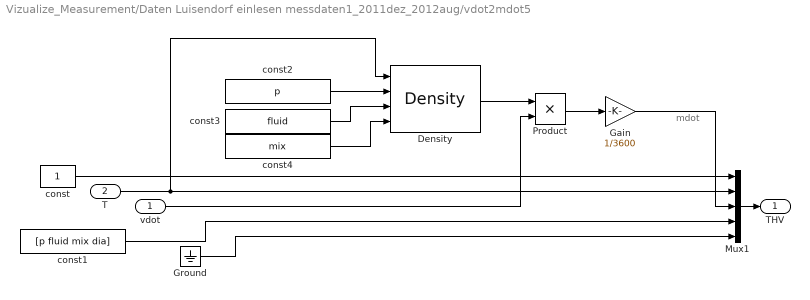
== system Vizualize_Measurement/Daten Luisendorf einlesen messdaten1_2011dez_2012aug/vdot2mdot5 ==
  note: mdot
  vdot : Inport
  T : Inport  Port=2
  Density : carnot/Basic/Material_Properties/Density  VariantControl=CarlibClassic  INPUTARGUMENTS=state variables (classic)  DEBUGLEVEL=DEBUGLEVEL  MAXTOTALWARNINGS=inf  MAXCONSECUTIVEWARNINGS=inf  WRITETOFILE=0  FILENAME='errors.txt'
      settings: SourceProductName=Carnot
  Gain : Gain  Gain=1/3600
  Ground : Ground
  Mux1 : Mux  Inputs=[1 1 1 4 13]
  Product : Product  RndMeth=Zero
  const : Constant
  const1 : Constant  Value=[p fluid mix dia]
  const2 : Constant  Value=p
  const3 : Constant  Value=fluid
  const4 : Constant  Value=mix
  THV : Outport  InitialOutput=0
  wires:
  Gain/1 -> Mux1/3
  const1/1 -> Mux1/4
  T/1 -> Density/1, Mux1/2
  Ground/1 -> Mux1/5
  const/1 -> Mux1/1
  Mux1/1 -> THV/1
  const2/1 -> Density/2
  const3/1 -> Density/3
  const4/1 -> Density/4
  Density/1 -> Product/1
  vdot/1 -> Product/2
  Product/1 -> Gain/1

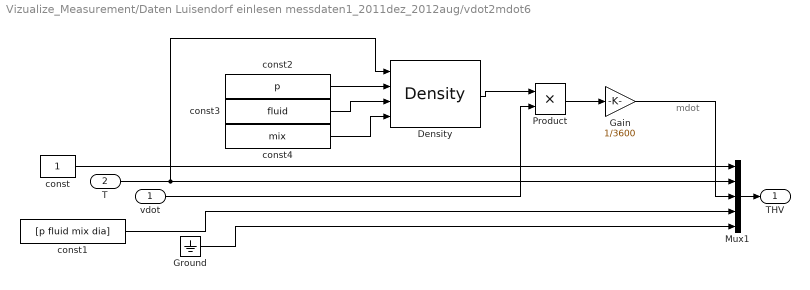
== system Vizualize_Measurement/Daten Luisendorf einlesen messdaten1_2011dez_2012aug/vdot2mdot6 ==
  note: mdot
  vdot : Inport
  T : Inport  Port=2
  Density : carnot/Basic/Material_Properties/Density  VariantControl=CarlibClassic  INPUTARGUMENTS=state variables (classic)  DEBUGLEVEL=DEBUGLEVEL  MAXTOTALWARNINGS=inf  MAXCONSECUTIVEWARNINGS=inf  WRITETOFILE=0  FILENAME='errors.txt'
      settings: SourceProductName=Carnot
  Gain : Gain  Gain=1/3600
  Ground : Ground
  Mux1 : Mux  Inputs=[1 1 1 4 13]
  Product : Product  RndMeth=Zero
  const : Constant
  const1 : Constant  Value=[p fluid mix dia]
  const2 : Constant  Value=p
  const3 : Constant  Value=fluid
  const4 : Constant  Value=mix
  THV : Outport  InitialOutput=0
  wires:
  Gain/1 -> Mux1/3
  const1/1 -> Mux1/4
  T/1 -> Density/1, Mux1/2
  Ground/1 -> Mux1/5
  const/1 -> Mux1/1
  Mux1/1 -> THV/1
  const2/1 -> Density/2
  const3/1 -> Density/3
  const4/1 -> Density/4
  Density/1 -> Product/1
  vdot/1 -> Product/2
  Product/1 -> Gain/1

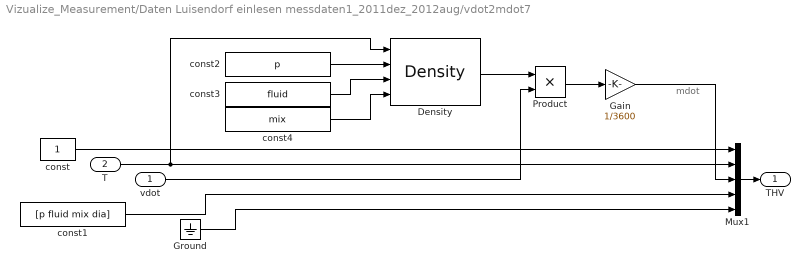
== system Vizualize_Measurement/Daten Luisendorf einlesen messdaten1_2011dez_2012aug/vdot2mdot7 ==
  note: mdot
  vdot : Inport
  T : Inport  Port=2
  Density : carnot/Basic/Material_Properties/Density  VariantControl=CarlibClassic  INPUTARGUMENTS=state variables (classic)  DEBUGLEVEL=DEBUGLEVEL  MAXTOTALWARNINGS=inf  MAXCONSECUTIVEWARNINGS=inf  WRITETOFILE=0  FILENAME='errors.txt'
      settings: SourceProductName=Carnot
  Gain : Gain  Gain=1/3600
  Ground : Ground
  Mux1 : Mux  Inputs=[1 1 1 4 13]
  Product : Product  RndMeth=Zero
  const : Constant
  const1 : Constant  Value=[p fluid mix dia]
  const2 : Constant  Value=p
  const3 : Constant  Value=fluid
  const4 : Constant  Value=mix
  THV : Outport  InitialOutput=0
  wires:
  Product/1 -> Gain/1
  vdot/1 -> Product/2
  Density/1 -> Product/1
  const4/1 -> Density/4
  const3/1 -> Density/3
  const2/1 -> Density/2
  Mux1/1 -> THV/1
  const/1 -> Mux1/1
  Ground/1 -> Mux1/5
  T/1 -> Density/1, Mux1/2
  const1/1 -> Mux1/4
  Gain/1 -> Mux1/3
